simulink model "hev_series"  (R2015b)
settings: Solver=VariableStepAuto  StartTime=0.0  StopTime=100  RelTol=1e-3
undefined symbols (not defined in the file): A, C, etha, f, g, lam, M, N, p, r, Vw
libraries: simulink x1
settings Model: Creator=ihong-gyu  LastModifiedBy=ihong-gyu

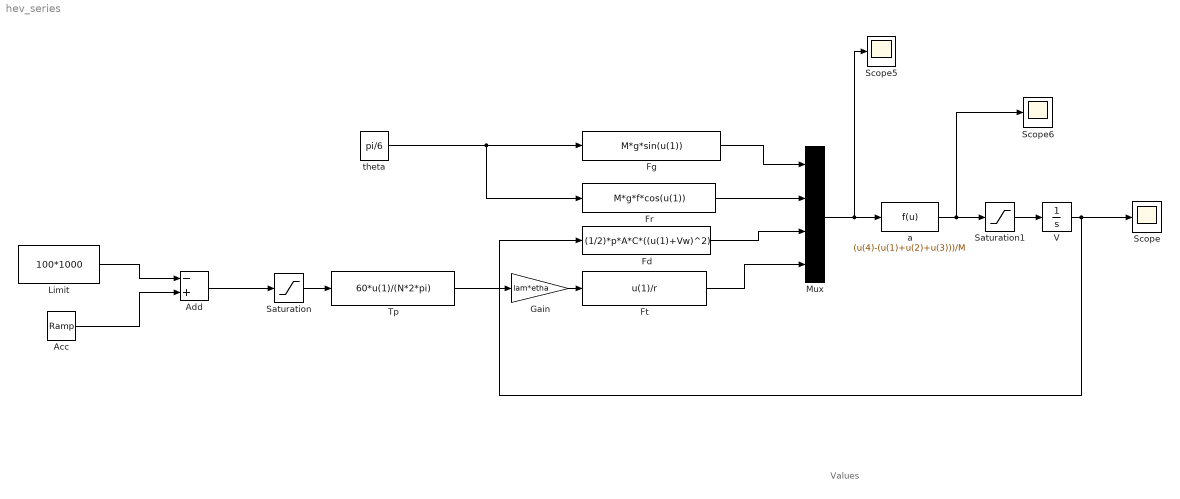
== system hev_series ==
  note: Values
  Acc : simulink/Sources/Ramp  slope=100*1000  start=0  X0=0
  Add : Sum  Inputs=-+
  Fd : Fcn  Expr=(1/2)*p*A*C*((u(1)+Vw)^2)
  Fg : Fcn  Expr=M*g*sin(u(1))
  Fr : Fcn  Expr=M*g*f*cos(u(1))
  Ft : Fcn  Expr=u(1)/r
  Gain : Gain  Gain=lam*etha
  Limit : Constant  Value=100*1000  SampleTime=8
  Mux : Mux
  Saturation : Saturate  UpperLimit=600*1000  LowerLimit=0
  Saturation1 : Saturate  UpperLimit=100000  LowerLimit=0
  Scope : Scope
  Scope5 : Scope
  Scope6 : Scope
  Tp : Fcn  Expr=60*u(1)/(N*2*pi)
  V : Integrator
  a : Fcn  Expr=(u(4)-(u(1)+u(2)+u(3)))/M
  theta : Constant  Value=pi/6
  wires:
  Fg/1 -> Mux/1
  Fr/1 -> Mux/2
  Fd/1 -> Mux/3
  Ft/1 -> Mux/4
  Mux/1 -> Scope5/1, a/1
  V/1 -> Fd/1, Scope/1
  theta/1 -> Fr/1, Fg/1
  a/1 -> Saturation1/1, Scope6/1
  Gain/1 -> Ft/1
  Tp/1 -> Gain/1
  Acc/1 -> Add/2
  Limit/1 -> Add/1
  Saturation/1 -> Tp/1
  Add/1 -> Saturation/1
  Saturation1/1 -> V/1
